simulink model "Pancake_FTC_Sam"  (Simulink 7.6)
settings: Solver=ode45  StartTime=0.0  StopTime=6000  MinStep=1e-5  RelTol=1e-3
InitFcn:
  | init;
StopFcn:
  | %plot_sim_result
  | save('SamSimResult.mat');
values from neighbouring files (symbols this model uses):
  m = length(Y_mat)/3    [PID_PD_4.m]    (also in Sam_FD.m = block.InputPort(2).Dimensions; myFD.m = block.OutputPort(1).Dimensions; myFD2.m = block.OutputPort(1).Dimensions; sys3.mat = 5)
  w = zeros(q,1)    [init.m]    (also in initMine.m; init_fd.m; plant_model.m = inp(2*n+m+1:2*n+m+q); plant_output.m = inp(2*n+m+1:2*n+m+q))
  x0 = zeros(2*n,1)    [init.m]    (also in initMine.m; init_fd.m = randn(2*n,1))
  yref = [1; 2; 0.5; -2; -3]    [init.m]    (also in initMine.m)
settings Model: Creator=Yao Hong Kok  LastModifiedBy=yaohong.kok
settings DebuggingCC: StrictBusMsg=Warning
settings SFSimCC: SimParseCustomCode=off

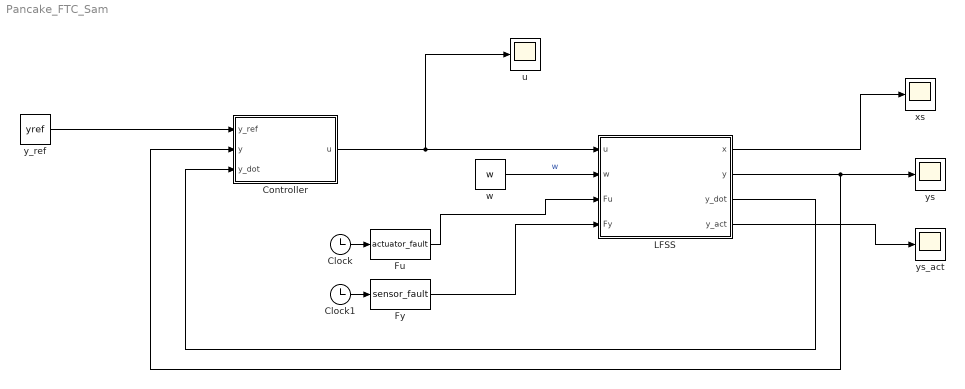
== system Pancake_FTC_Sam ==
  Clock : Clock
      settings: Decimation=10
  Clock1 : Clock
      settings: Decimation=10
  Controller : Subsystem
  Fu : MATLABFcn  MATLABFcn=actuator_fault
  Fy : MATLABFcn  MATLABFcn=sensor_fault
  LFSS : Subsystem
  u : Scope
      settings: SaveName=us
  w : Constant  Value=w
  xs : Scope
      settings: SaveName=xs
  y_ref : Constant  Value=yref
  ys : Scope
      settings: YMin=-400  YMax=250  SaveName=ys
  ys_act : Scope
      settings: YMax=27.5  SaveName=ys4
  wires:
  LFSS/1(x) -> xs/1
  LFSS/2(y) -> ys/1, Controller/2(y)
  w/1 -> LFSS/2(w)  "w"
  Clock/1 -> Fu/1
  Fu/1 -> LFSS/3(Fu)
  Clock1/1 -> Fy/1
  Fy/1 -> LFSS/4(Fy)
  Controller/1(u) -> LFSS/1(u), u/1
  y_ref/1 -> Controller/1(y_ref)
  LFSS/3(y_dot) -> Controller/3(y_dot)
  LFSS/4(y_act) -> ys_act/1

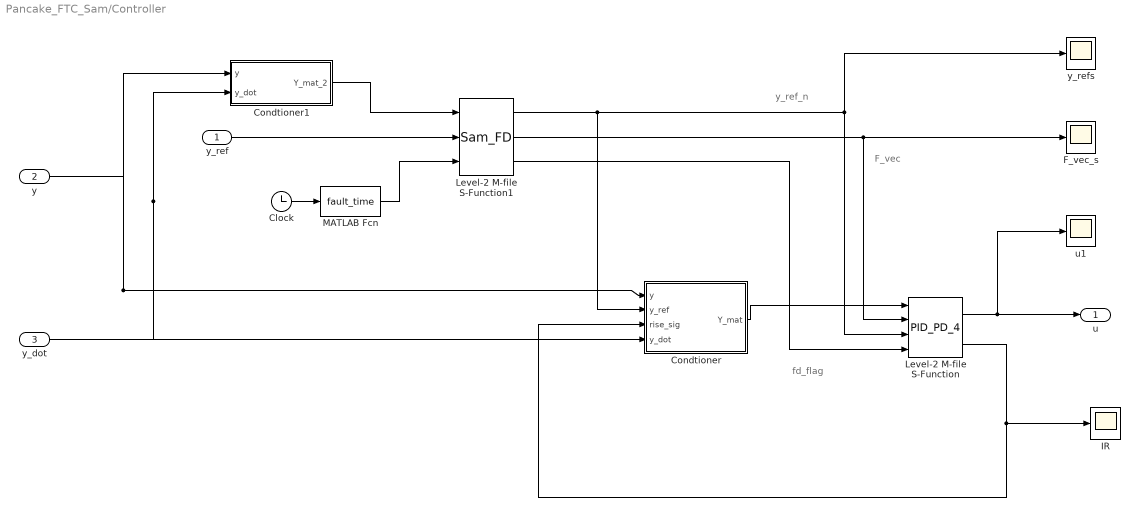
== system Pancake_FTC_Sam/Controller ==
  note: y_ref_n
  note: F_vec
  note: fd_flag
  y_ref : Inport
  y : Inport  Port=2
  y_dot : Inport  Port=3
  Clock : Clock
      settings: Decimation=10
  Condtioner : Subsystem
  Condtioner1 : Subsystem
  F_vec_s : Scope
      settings: SaveName=F_vec_s
  IR : Scope
      settings: SaveName=ys1
  Level-2 M-file S-Function : M-S-Function  FunctionName=PID_PD_4
  Level-2 M-file S-Function1 : M-S-Function  FunctionName=Sam_FD
  MATLAB Fcn : MATLABFcn  MATLABFcn=fault_time
  u1 : Scope
      settings: SaveName=ys3
  y_refs : Scope
      settings: SaveName=y_ref_s
  u : Outport
  wires:
  Condtioner/1(Y_mat) -> Level-2 M-file S-Function/1
  Level-2 M-file S-Function/1 -> u/1, u1/1
  y/1 -> Condtioner/1(y), Condtioner1/1(y)
  y_ref/1 -> Level-2 M-file S-Function1/2
  Level-2 M-file S-Function/2 -> Condtioner/3(rise_sig), IR/1
  Level-2 M-file S-Function1/1 -> Level-2 M-file S-Function/3, y_refs/1, Condtioner/2(y_ref)
  Level-2 M-file S-Function1/2 -> Level-2 M-file S-Function/2, F_vec_s/1
  Level-2 M-file S-Function1/3 -> Level-2 M-file S-Function/4
  MATLAB Fcn/1 -> Level-2 M-file S-Function1/3
  Clock/1 -> MATLAB Fcn/1
  Condtioner1/1(Y_mat_2) -> Level-2 M-file S-Function1/1
  y_dot/1 -> Condtioner1/2(y_dot), Condtioner/4(y_dot)

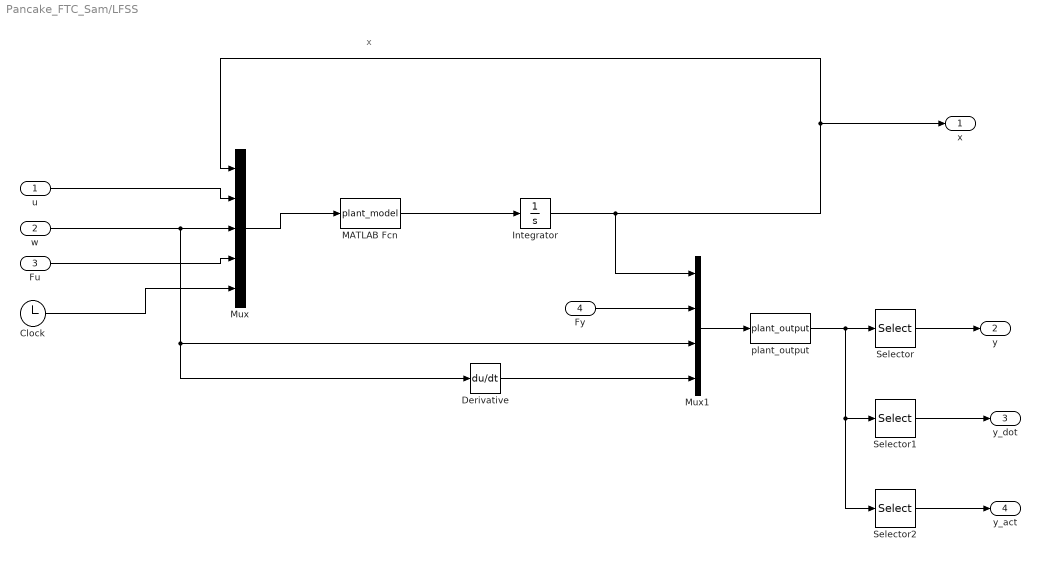
== system Pancake_FTC_Sam/LFSS ==
  note: x
  u : Inport
  w : Inport  Port=2
  Fu : Inport  Port=3
  Fy : Inport  Port=4
  Clock : Clock
  Derivative : Derivative
  Integrator : Integrator  InitialCondition=x0
  MATLAB Fcn : MATLABFcn  MATLABFcn=plant_model
  Mux : Mux  Inputs=5
  Mux1 : Mux
  Selector : Selector  InputPortWidth=3*m  IndexOptions=Index vector (dialog)  Indices=[1:m]  OutputSizes=1
  Selector1 : Selector  InputPortWidth=3*m  IndexOptions=Index vector (dialog)  Indices=[m+1:2*m]  OutputSizes=1
  Selector2 : Selector  InputPortWidth=3*m  IndexOptions=Index vector (dialog)  Indices=[2*m+1:3*m]  OutputSizes=1
  plant_output : MATLABFcn  MATLABFcn=plant_output
  x : Outport
  y : Outport  Port=2
  y_dot : Outport  Port=3
  y_act : Outport  Port=4
  wires:
  MATLAB Fcn/1 -> Integrator/1
  Mux/1 -> MATLAB Fcn/1
  Integrator/1 -> Mux/1, x/1, Mux1/1
  u/1 -> Mux/2
  w/1 -> Mux/3, Mux1/3, Derivative/1
  Fu/1 -> Mux/4
  Mux1/1 -> plant_output/1
  Fy/1 -> Mux1/2
  Clock/1 -> Mux/5
  Derivative/1 -> Mux1/4
  plant_output/1 -> Selector/1, Selector1/1, Selector2/1
  Selector/1 -> y/1
  Selector1/1 -> y_dot/1
  Selector2/1 -> y_act/1

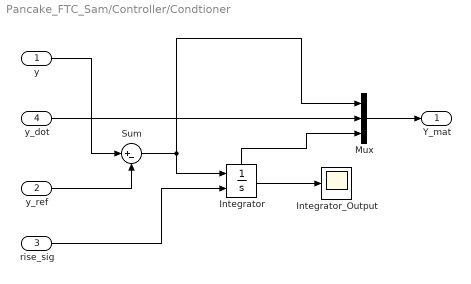
== system Pancake_FTC_Sam/Controller/Condtioner ==
  y : Inport
  y_ref : Inport  Port=2
  rise_sig : Inport  Port=3
  y_dot : Inport  Port=4
  Integrator : Integrator  ExternalReset=either  ShowStatePort=on
  Integrator_Output : Scope
      settings: SaveName=ys2
  Mux : Mux  Inputs=3
  Sum : Sum  Inputs=|+-
  Y_mat : Outport
  wires:
  Mux/1 -> Y_mat/1
  y/1 -> Sum/1
  y_ref/1 -> Sum/2
  Sum/1 -> Integrator/1, Mux/1
  rise_sig/1 -> Integrator/2
  Integrator/State -> Mux/3
  Integrator/1 -> Integrator_Output/1
  y_dot/1 -> Mux/2

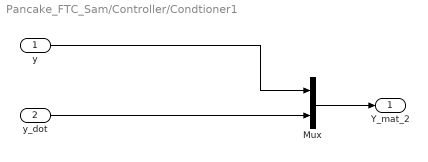
== system Pancake_FTC_Sam/Controller/Condtioner1 ==
  y : Inport
  y_dot : Inport  Port=2
  Mux : Mux  Inputs=2
  Y_mat_2 : Outport
  wires:
  Mux/1 -> Y_mat_2/1
  y/1 -> Mux/1
  y_dot/1 -> Mux/2
